simulink model "Multicopter_vPC"  (R2017b)
settings: Solver=ode4  StartTime=0.0  StopTime=inf  FixedStep=0.0002  RelTol=1e-3
values from neighbouring files (symbols this model uses):
  ModelFailBatt_CustomHovTime = 15    [Init.m]
  ModelFailBatt_isEnable = boolean(0)    [Init.m]
  ModelFailBatt_islowCapacity = boolean(0)    [Init.m]
  ModelFailBatt_isLowVoltage = boolean(0)    [Init.m]
  ModelFailBatt_isPowOff = boolean(0)    [Init.m]
  ModelFailBatt_isUseCustomHovTime = boolean(0)    [Init.m]
  ModelFailBatt_remainCapacityRatio = 0.2    [Init.m]
  ModelFailBatt_remainVoltageRatio = 0.5    [Init.m]
  ModelFailEnable = boolean(0)    [Init.m]
  ModelFailLoad_isEnable = boolean(0)    [Init.m]
  ModelFailLoad_isLoadFall = boolean(0)    [Init.m]
  ModelFailLoad_isLoadLeak = boolean(0)    [Init.m]
  ModelFailLoad_isLoadShift = boolean(0)    [Init.m]
  ModelFailLoad_LoadLeakRatioRate = 0    [Init.m]
  ModelFailLoad_loadMassRatio = 0    [Init.m]
  ModelFailLoad_LoadShiftXRatio = 0    [Init.m]
  ModelFailLoad_LoadShiftYRatio = 0    [Init.m]
  ModelFailLoad_LoadShiftZRatio = 0    [Init.m]
  ModelFailProp_isEnable = boolean(1)    [Init.m]
  ModelFailProp_PropEffRatioVec = ones(1,8)    [Init.m]
  ModelFailWind_ConstWindX = 0    [Init.m]
  ModelFailWind_ConstWindY = 0    [Init.m]
  ModelFailWind_ConstWindZ = 0    [Init.m]
  ModelFailWind_GustWindFreq = 0    [Init.m]
  ModelFailWind_GustWindStrength = 0    [Init.m]
  ModelFailWind_isConstWind = boolean(0)    [Init.m]
  ModelFailWind_isEnable = boolean(0)    [Init.m]
  ModelFailWind_isGustWind = boolean(0)    [Init.m]
  ModelFailWind_isSheerWind = boolean(0)    [Init.m]
  ModelFailWind_isTurbWind = boolean(0)    [Init.m]
  ModelFailWind_SheerWindDirec = 0    [Init.m]
  ModelFailWind_SheerWindStrength = 0    [Init.m]
  ModelFailWind_TurbWindDirec = 0    [Init.m]
  ModelFailWind_TurbWindStrength = 0    [Init.m]
  ModelInit_RPM = 0    [Init.m]
  ModelParam_BattHoverMinutes = 18    [Init.m]
  ModelParam_BattHoverThr = 0.609    [Init.m]
  ModelParam_envAltitude = -41.5260009765625    (= -41.5260009766)    [Init.m]
  ModelParam_GlobalNoiseGainSwitch = 0    [Init.m]
  ModelParam_GPSEphFinal = 0.3    [Init.m]
  ModelParam_GPSEpvFinal = 0.4    [Init.m]
  ModelParam_GPSFix3DFix = 3    [Init.m]
  ModelParam_GPSSatsVisible = 10    [Init.m]
  ModelParam_motorCr = 1148    [Init.m]
  ModelParam_motorJm = 0.0001287    [Init.m]
  ModelParam_motorMinThr = 0.05    [Init.m]
  ModelParam_motorT = 0.02    [Init.m]
  ModelParam_motorWb = -141.4    [Init.m]
  ModelParam_noiseBaroCoupleWithSpeed = 0    [Init.m]
  ModelParam_noiseGPSSampTime = 0.2    [Init.m]
  ModelParam_noisePowerIMU = 0    [Init.m]
  ModelParam_noisePowerOffGainAccel = 0.04    [Init.m]
  ModelParam_noisePowerOffGainAccelZ = 0.03    [Init.m]
  ModelParam_noisePowerOffGainGyro = 0.02    [Init.m]
  ModelParam_noisePowerOffGainGyroZ = 0.025    [Init.m]
  ModelParam_noisePowerOffGainMag = 0.02    [Init.m]
  ModelParam_noisePowerOffGainMagZ = 0.035    [Init.m]
  ModelParam_noisePowerOnGainAccel = 0.8    [Init.m]
  ModelParam_noisePowerOnGainAccelZ = 4.5    [Init.m]
  ModelParam_noisePowerOnGainGyro = 2    [Init.m]
  ModelParam_noisePowerOnGainGyroZ = 1    [Init.m]
  ModelParam_noisePowerOnGainMag = 0.025    [Init.m]
  ModelParam_noisePowerOnGainMagZ = 0.05    [Init.m]
  ModelParam_noiseSampleTimeAccel = 0.001    [Init.m]
  ModelParam_noiseSampleTimeGyro = 0.001    [Init.m]
  ModelParam_noiseSampleTimeMag = 0.01    [Init.m]
  ModelParam_noiseUpperBaro = 0    [Init.m]
  ModelParam_noiseUpperGPS = 0.5    [Init.m]
  ModelParam_noiseUpperWindBodyRatio = 0    [Init.m]
  ModelParam_noiseWindSampTime = 0.001    [Init.m]
  ModelParam_rotorCm = 1.779e-07    [Init.m]
  ModelParam_rotorCt = 1.105e-05    [Init.m]
  ModelParam_timeSampBaro = 0.01    [Init.m]
  ModelParam_uavCCm = [0.0035 0.0039 0.0034]    [Init.m]
  ModelParam_uavCd = 0.055    [Init.m]
  ModelParam_uavDearo = 0.12    [Init.m]
  ModelParam_uavJ = [ModelParam_uavJxx,0,0;     0,ModelParam_uavJyy,0;     0,0,ModelParam_uavJzz]    [Init.m]
  ModelParam_uavMass = 1.4    [Init.m]
  ModelParam_uavMotNumbs = int8(4)    [Init.m]
  ModelParam_uavR = 0.225    [Init.m]
  ModelParam_uavType = int8(3)    [Init.m]
undefined symbols (not defined in the file or in its folder): d_i, Earth, F, h_i, Light, MIL, ModelParam_GPSEphInitial, ModelParam_GPSEphTimeConstant, ModelParam_GPSEpvInitial, ModelParam_GPSEpvTimeConstant, ModelParam_noiseLowPassFilterCoeAccel, ModelParam_noiseLowPassFilterCoeGyro, ModelParam_timeSamp, Moderate, Newton, Raphson, WGS84
libraries: simulink x12, aerolibasang x4, aerolibwind2 x3, aerolibtransform2 x3, sharedtransform x3, aerolibutil x2, sharedutil x2, shared6dof x1, aerolibatmos2 x1, aerolibconvert2 x1, aerolibobsolete x1, aerolibnav x1
(part 3 of 3)

== matlab function Multicopter_vPC/Force and Moment Model/Body AeroCenter ==
  data: Fd output; Md output; wb input; Vb input; Cd input; CCm input; uavDearo input
function [Fd,Md] = fcn(wb,Vb,Cd, CCm, uavDearo)
% This is control effectiveness model, where Fb is the force produced by motors, Mb is
% the moment produced by motors, and Fd is the resistance produced by the air.
% The gyroscopic torque is not considered here.
% uavDearo 机身重心位置，向下为正

 Fd = -Cd*Vb.*abs(Vb);%
 
 Mfd=[Fd(2)*uavDearo;-Fd(1)*uavDearo;0];
 
Md=-CCm.*wb.*abs(wb);
Md=Mfd+Md;
%  CCm=4.72e-3;
%  Md=-CCm*wb.*abs(wb)*0.5;%0.3
%  Md= Mfd+Md;
 
end

== matlab function Multicopter_vPC/OutputPort/HILSensorMavModel/MotorNoiseScaleCoe ==
  data: PWMin input; NoiseScaleCoe output
function NoiseScaleCoe = fcn(PWMin)
%本函数输一个分段函数，分为三段三段斜率不同，具体形状可以通过修改下面四个参数设置

%如何设置合理参数使得噪声在此分段函数前提下更加真实  
%1、首先采集实际飞行过程中飞机的噪声水平然后修改噪声模块的幅值
%2、飞机静止时的噪声则可以通过设置keyPoint1的数值，也就是本分段函数的自变量值为0时候的函数值来调整静止时候飞机传感器噪声

%分段函数有两个起点和转折点，下面四个点一次对应起点两个拐点终点，第一个数表示和坐标的数值，第二个表示对应的函数值
%默认  输入为1是函数值也是1
keyPoint1 = [0 0.05];%不要修改 数字0
keyPoint2 = [0.8 1];
keyPoint3 = [1.7 1];
keyPoint4 = [2 2];%不要修改

%m 范围 0-2 50%油门时候为 m = 1
m = 2*mean(PWMin);
if m <keyPoint2(1)
    NoiseScaleCoe = ((keyPoint2(2) - keyPoint1(2))/(keyPoint2(1)-keyPoint1(1)))*(m - keyPoint1(1)) + keyPoint1(2);
else
    if m > keyPoint2(1) && m < keyPoint3(1)
        NoiseScaleCoe = ((keyPoint3(2) - keyPoint2(2))/(keyPoint3(1)-keyPoint2(1)))*(m - keyPoint2(1)) + keyPoint2(2);
    else
        NoiseScaleCoe = ((keyPoint4(2) - keyPoint3(2))/(keyPoint4(1)-keyPoint3(1)))*(m - keyPoint3(1)) + keyPoint3(2);
    end
end
